simulink model "testing"  (R2017a)
settings: Solver=VariableStepAuto  StartTime=0.0  StopTime=10  RelTol=1e-3
values from neighbouring files (symbols this model uses):
  Atest = [0 1;0 0]    [testing_linear_observer.m]
  Btest = [0;1]    [testing_linear_observer.m]
  Ctest = [1 0]    [testing_linear_observer.m]
  KKK = place(Aaug,Baug,desired_vp_i)    [testing_linear_observer.m]
  L = [3 1]'    [Non_linear_observers_.m]    (also in projet_AAV.m = 1; testing_linear_observer.m = L')
settings Model: Creator=firass2019  LastModifiedBy=firass2019

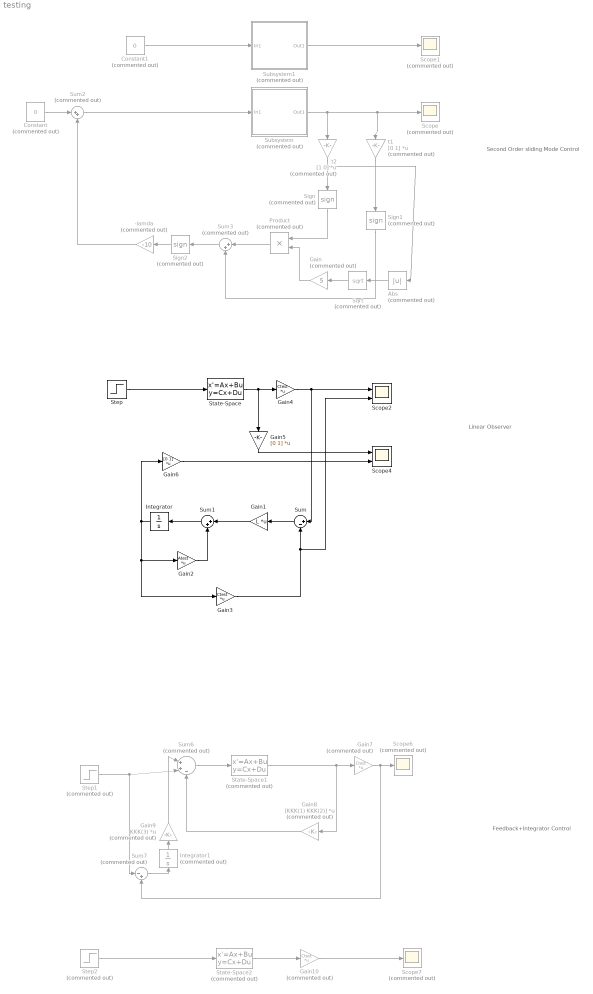
== system testing ==
  note: Feedback+Integrator Control
  note: Linear Observer
  note: Second Order sliding Mode Control
  -lamda : Gain  Commented=on  Gain=-10
  Abs : Abs  Commented=on
  Constant : Constant  Commented=on  Value=0
  Constant1 : Constant  Commented=on  Value=0
  Gain : Gain  Commented=on  Gain=5
  Gain1 : Gain  Gain=L  Multiplication=Matrix(K*u)
  Gain10 : Gain  Commented=on  Gain=Ctest  Multiplication=Matrix(K*u)
  Gain2 : Gain  Gain=Atest  Multiplication=Matrix(K*u)
  Gain3 : Gain  Gain=Ctest  Multiplication=Matrix(K*u)
  Gain4 : Gain  Gain=Ctest  Multiplication=Matrix(K*u)
  Gain5 : Gain  Gain=[0 1]  Multiplication=Matrix(K*u)
  Gain6 : Gain  Gain=[0 1]  Multiplication=Matrix(K*u)
  Gain7 : Gain  Commented=on  Gain=Ctest  Multiplication=Matrix(K*u)
  Gain8 : Gain  Commented=on  Gain=[KKK(1) KKK(2)]  Multiplication=Matrix(K*u)
  Gain9 : Gain  Commented=on  Gain=KKK(3)  Multiplication=Matrix(K*u)
  Integrator : Integrator
  Integrator1 : Integrator  Commented=on
  Product : Product  Commented=on
  Scope{,1,6..7} (4 alike) : Scope  Commented=on
  Scope2 : Scope  NumInputPorts=2
  Scope4 : Scope  NumInputPorts=2
  Sign : Signum  Commented=on  ZeroCross=off
  Sign1 : Signum  Commented=on  ZeroCross=off
  Sign2 : Signum  Commented=on  ZeroCross=off
  Sqrt : Sqrt  Commented=on  SaturateOnIntegerOverflow=on
  State-Space : StateSpace  A=Atest  B=Btest  C=[1 0;0 1]  D=[0 ;0 ]  X0=[5;0]
  State-Space1 : StateSpace  Commented=on  A=Atest  B=Btest  C=[1 0;0 1]  D=[0 ;0 ]  X0=[0;0]
  State-Space2 : StateSpace  Commented=on  A=Atest  B=Btest  C=[1 0;0 1]  D=[0 ;0 ]  X0=[0;0]
  Step : Step  Time=0  SampleTime=0
  Step1 : Step  Commented=on  Time=0  SampleTime=0
  Step2 : Step  Commented=on  Time=0  SampleTime=0
  Subsystem : Subsystem  Commented=on
  Subsystem1 : Subsystem  Commented=on
  Sum : Sum  Inputs=|+-
  Sum1 : Sum  Inputs=|++
  Sum2 : Sum  Commented=on  Inputs=|++
  Sum3 : Sum  Commented=on  Inputs=|++
  Sum6 : Sum  Commented=on  Inputs=|++-
  Sum7 : Sum  Commented=on  Inputs=|-+
  t1 : Gain  Commented=on  Gain=[0 1]  Multiplication=Matrix(K*u)
  t2 : Gain  Commented=on  Gain=[1 0]  Multiplication=Matrix(K*u)
  wires:
  t2/1 -> Abs/1, Sign/1
  t1/1 -> Sign1/1
  Constant/1 -> Sum2/1
  Sum2/1 -> Subsystem/1(In1)
  Constant1/1 -> Subsystem1/1(In1)
  Subsystem1/1(Out1) -> Scope1/1
  Sign1/1 -> Sum3/2
  Sign/1 -> Product/1
  Abs/1 -> Sqrt/1
  Sqrt/1 -> Gain/1
  Gain/1 -> Product/2
  Product/1 -> Sum3/1
  Sum3/1 -> Sign2/1
  Sign2/1 -> -lamda/1
  -lamda/1 -> Sum2/2
  Subsystem/1(Out1) -> t2/1, Scope/1, t1/1
  Step/1 -> State-Space/1
  State-Space/1 -> Gain5/1, Gain4/1
  Sum/1 -> Gain1/1
  Gain1/1 -> Sum1/1
  Gain2/1 -> Sum1/2
  Integrator/1 -> Gain2/1, Gain3/1, Gain6/1
  Gain3/1 -> Sum/2, Scope2/2
  Sum1/1 -> Integrator/1
  Gain4/1 -> Scope2/1, Sum/1
  Gain5/1 -> Scope4/1
  Gain6/1 -> Scope4/2
  State-Space1/1 -> Gain7/1, Gain8/1
  Gain7/1 -> Sum7/2, Scope6/1
  Step1/1 -> Sum7/1, Sum6/2
  Sum6/1 -> State-Space1/1
  Gain8/1 -> Sum6/3
  Gain9/1 -> Sum6/1
  Integrator1/1 -> Gain9/1
  Sum7/1 -> Integrator1/1
  Step2/1 -> State-Space2/1
  Gain10/1 -> Scope7/1
  State-Space2/1 -> Gain10/1

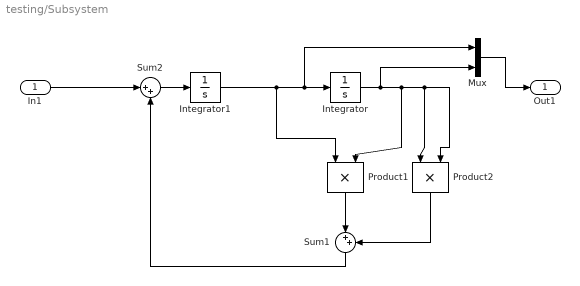
== system testing/Subsystem ==
  In1 : Inport
  Integrator : Integrator  InitialCondition=0.5
  Integrator1 : Integrator
  Mux : Mux  Inputs=2
  Product1 : Product
  Product2 : Product
  Sum1 : Sum  Inputs=|++
  Sum2 : Sum  Inputs=|++
  Out1 : Outport
  wires:
  Sum2/1 -> Integrator1/1
  Sum1/1 -> Sum2/2
  In1/1 -> Sum2/1
  Integrator1/1 -> Product1/1, Mux/1, Integrator/1
  Product2/1 -> Sum1/2
  Product1/1 -> Sum1/1
  Integrator/1 -> Mux/2, Product1/2, Product2/2, Product2/1
  Mux/1 -> Out1/1

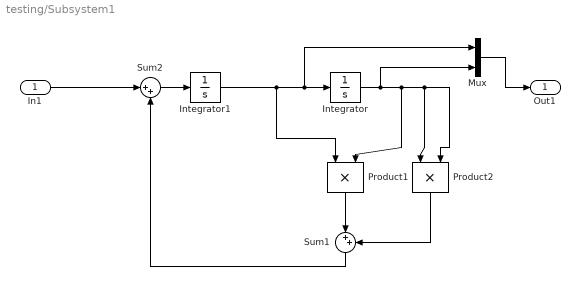
== system testing/Subsystem1 ==
  In1 : Inport
  Integrator : Integrator  InitialCondition=0.1
  Integrator1 : Integrator
  Mux : Mux  Inputs=2
  Product1 : Product
  Product2 : Product
  Sum1 : Sum  Inputs=|++
  Sum2 : Sum  Inputs=|++
  Out1 : Outport
  wires:
  Mux/1 -> Out1/1
  Integrator/1 -> Product2/1, Product2/2, Product1/2, Mux/2
  Product1/1 -> Sum1/1
  Product2/1 -> Sum1/2
  Integrator1/1 -> Integrator/1, Mux/1, Product1/1
  In1/1 -> Sum2/1
  Sum1/1 -> Sum2/2
  Sum2/1 -> Integrator1/1
